simulink model "P7"  (R2022b)
settings: Solver=VariableStepAuto  StartTime=0.0  StopTime=10.0  RelTol=1e-3
settings Model: Creator=osvid  LastModifiedBy=andre

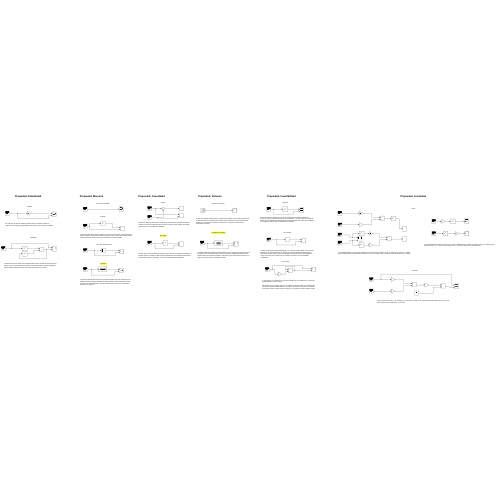
[thumbnail: Simulink's stored preview of the top-level diagram]
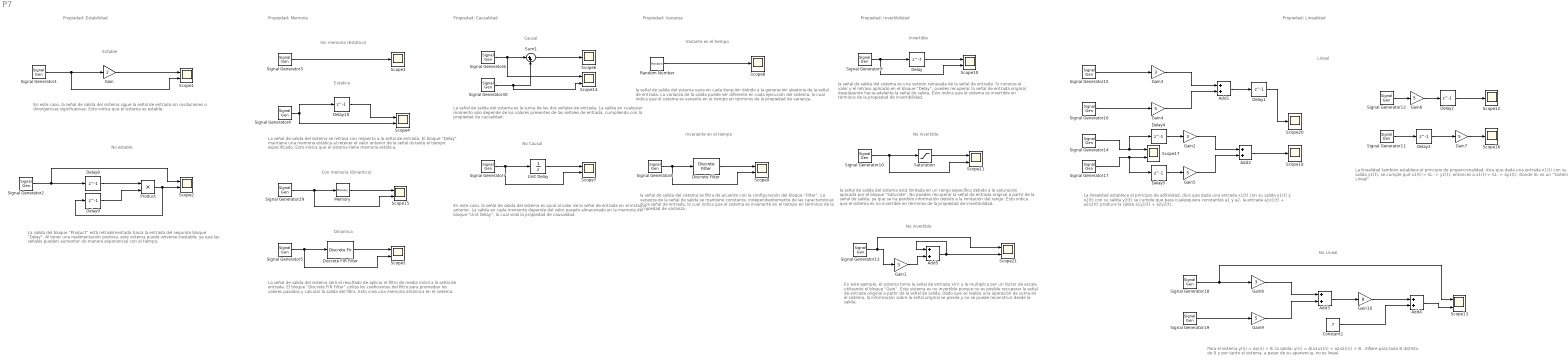
== system P7 ==
  note: la señal de salida del sistema está limitada en un rango específico debido a la saturación aplicada por el bloque "Saturate". No puedes recuperar la señal de entrada original a partir de la señal de salida, ya que se ha perdido información debido a la limitación del rango. Esto indica que el sistema es no invertible en términos de la propiedad de invertibilidad.
  note: la señal de salida del sistema es una versión retrasada de la señal de entrada. Si conoces el valor y el retraso aplicado en el bloque "Delay", puedes recuperar la señal de entrada original desplazando hacia adelante la señal de salida. Esto indica que el sistema es invertible en términos de la propiedad de invertibilidad.
  note: Invertible
  note: la señal de salida del sistema se filtra de acuerdo con la configuración del bloque "Filter". La varianza de la señal de salida se mantiene constante, independientemente de las características de la señal de entrada, lo cual indica que el sistema es invariante en el tiempo en términos de la propiedad de varianza.
  note: la señal de salida del sistema varía en cada iteración debido a la generación aleatoria de la señal de entrada. La varianza de la salida puede ser diferente en cada ejecución del sistema, lo cual indica que el sistema es variante en el tiempo en términos de la propiedad de varianza.
  note: En este caso, la señal de salida del sistema es igual al valor de la señal de entrada en el instante anterior. La salida en cada momento depende del valor pasado almacenado en la memoria del bloque "Unit Delay", lo cual viola la propiedad de causalidad.
  note: Causal
  note: La señal de salida del sistema es la suma de las dos señales de entrada. La salida en cualquier momento solo depende de los valores presentes de las señales de entrada, cumpliendo con la propiedad de causalidad.
  note: La señal de salida del sistema será el resultado de aplicar el filtro de media móvil a la señal de entrada. El bloque "Discrete FIR Filter" utiliza los coeficientes del filtro para promediar los valores pasados y calcular la salida del filtro. Esto crea una memoria dinámica en el sistema.
  note: La señal de salida del sistema se retrasa con respecto a la señal de entrada. El bloque "Delay" mantiene una memoria estática al retener el valor anterior de la señal durante el tiempo especificado. Esto indica que el sistema tiene memoria estática.
  note: En este caso, la señal de salida del sistema sigue la señal de entrada sin oscilaciones o divergencias significativas. Esto indica que el sistema es estable.
  note: La salida del bloque "Product" está retroalimentada hacia la entrada del segundo bloque "Delay". Al tener una realimentación positiva, este sistema puede volverse inestable, ya que las señales pueden aumentar de manera exponencial con el tiempo.
  note: Invariante en el tiempo
  note: Dinamica
  note: Sin memoria (Estatico)
  note: No estable
  note: Propiedad: Memoria
  note: Estable
  note: Propiedad: Estabilidad
  note: Estatica
  note: Propiedad: Causalidad
  note: Propiedad: Varianza
  note: Variante en el tiempo
  note: Propiedad: Invertibilidad
  note: Con memoria (Dinamico)
  note: No Causal
  note: Propiedad: Linealidad
  note: No invertible
  note: Lineal
  note: La linealidad establece el principio de aditividad, dice que dada una entrada x1(t) con su salida y1(t) y x2(t) con su salida y2(t) se cumple qué para cualesquiera constantes a1 y a2, la entrada a1x1(t) + a2x2(t) produce la salida a1y1(t) + a2y2(t).
  note: No Lineal
  note: La linealidad también establece el principio de proporcionalidad, dice que dada una entrada x1(t) con su salida y1(t), se cumple qué x1(t)-> SL -> y1(t), entonces a x1(t)-> SL -> ay1(t). Donde SL es un "Sistema Lineal"
  note: Para el sistema y(n) = Ax(n) + B, la salida: y(n) = A(a1x1(n) + a2x2(n)) + B , difiere para todo B distinto de 0 y por tanto el sistema, a pesar de su apariencia, no es lineal.
  note: En este ejemplo, el sistema toma la señal de entrada x(n) y la multiplica por un factor de escala utilizando el bloque "Gain".
      | Este sistema es no invertible porque no es posible recuperar la señal de entrada original a partir de la señal de salida. Dado que se realiza una operación de suma en el sistema, la información sobre la señal original se pierde y no se puede reconstruir desde la salida.
  note: No invertible
  Add{1..5} (5 alike) : Sum
  Constant1 : Constant  Value=7
  Delay : Delay  DelayLength=7  InitialCondition=0
  Delay{1..5,8..10} (8 alike) : Delay  DelayLength=1  InitialCondition=0
  Discrete FIR Filter : DiscreteFir
  Discrete Filter : DiscreteFilter
  Gain : Gain  Gain=2
  Gain{1,4..7,9} (6 alike) : Gain  Gain=5
  Gain10 : Gain  Gain=8
  Gain2 : Gain  Gain=3
  Gain3 : Gain  Gain=3
  Gain8 : Gain  Gain=3
  Memory : Memory
  Product : Product
  Random Number : RandomNumber  SampleTime=0.1
  Saturation : Saturate
  Scope{1..2,4..5,7,9..11,13..15,17,21} (13 alike) : Scope  NumInputPorts=2
  Scope{3,6,8,12,16,18,20} (7 alike) : Scope
  Signal Generator{1..10,13,18..19,29} (14 alike) : SignalGenerator  Units=rad/sec
  Signal Generator{11..12,14..17,30} (7 alike) : SignalGenerator  WaveForm=square  Units=rad/sec
  Sum1 : Sum  Inputs=|++
  Unit Delay : UnitDelay  SampleTime=-1  HasFrameUpgradeWarning=on
  wires:
  Signal Generator1/1 -> Scope1/2, Gain/1
  Gain/1 -> Scope1/1
  Signal Generator3/1 -> Scope3/1
  Signal Generator5/1 -> Discrete FIR Filter/1, Scope5/2
  Signal Generator4/1 -> Delay10/1, Scope4/2
  Delay10/1 -> Scope4/1
  Discrete FIR Filter/1 -> Scope5/1
  Signal Generator29/1 -> Scope15/2, Memory/1
  Memory/1 -> Scope15/1
  Signal Generator6/1 -> Scope14/1, Sum1/1
  Signal Generator30/1 -> Scope14/2, Sum1/2
  Sum1/1 -> Scope6/1
  Signal Generator7/1 -> Scope7/2, Unit Delay/1
  Unit Delay/1 -> Scope7/1
  Random Number/1 -> Scope8/1
  Signal Generator8/1 -> Scope9/2, Discrete Filter/1
  Discrete Filter/1 -> Scope9/1
  Signal Generator9/1 -> Scope10/2, Delay/1
  Delay/1 -> Scope10/1
  Signal Generator10/1 -> Scope11/2, Saturation/1
  Saturation/1 -> Scope11/1
  Signal Generator16/1 -> Gain4/1
  Signal Generator15/1 -> Gain3/1
  Gain3/1 -> Add1/1
  Gain4/1 -> Add1/2
  Gain5/1 -> Add2/2
  Signal Generator14/1 -> Delay4/1, Scope17/1
  Signal Generator17/1 -> Delay5/1, Scope17/2
  Gain2/1 -> Add2/1
  Add2/1 -> Scope18/1
  Delay2/1 -> Scope12/1
  Signal Generator11/1 -> Delay3/1
  Signal Generator12/1 -> Gain6/1
  Gain6/1 -> Delay2/1
  Delay3/1 -> Gain7/1
  Gain7/1 -> Scope16/1
  Add1/1 -> Delay1/1
  Delay1/1 -> Scope20/1
  Delay4/1 -> Gain2/1
  Delay5/1 -> Gain5/1
  Signal Generator2/1 -> Scope2/1, Delay8/1
  Product/1 -> Delay9/1, Scope2/2
  Delay8/1 -> Product/1
  Delay9/1 -> Product/2
  Signal Generator18/1 -> Scope13/1, Gain8/1
  Gain9/1 -> Add3/2
  Signal Generator19/1 -> Gain9/1
  Gain8/1 -> Add3/1
  Add3/1 -> Gain10/1
  Constant1/1 -> Add4/2
  Gain10/1 -> Add4/1
  Add4/1 -> Scope13/2
  Signal Generator13/1 -> Scope21/1, Gain1/1
  Gain1/1 -> Add5/2
  Add5/1 -> Add5/1, Scope21/2
